simulink model "MDCC_DeadComp"  (R2023a)
settings: Solver=FixedStepDiscrete  StartTime=0.0  StopTime=10.0  FixedStep=0.0001  RelTol=1e-3
model workspace (MATLAB code in the model file):
  | cmdLim = Simulink.Parameter;
  | cmdLim.Value = 15;
  | cmdLim.Description = 'Limit for controlling the maximum surface command angle.';
  | cmdLim.Min = 0;
  | cmdLim.Max = 90;
  | cmdLim.DocUnits = 'deg';
  | 
  | dispGain = Simulink.Parameter;
  | dispGain.Value = 0.75;
  | dispGain.Description = 'Gain applied to the displacement error.';
  | dispGain.Min = 0;
  | dispGain.Max = [];
  | dispGain.DocUnits = 'deg/sec/deg';
  | 
  | dispLim = Simulink.Parameter;
  | dispLim.Value = 30;
  | dispLim.Description = 'Limit for controlling the maximum commanded angle.';
  | dispLim.Min = 0;
  | dispLim.Max = 180;
  | dispLim.DocUnits = 'deg';
  | 
  | intGain = Simulink.Parameter;
  | intGain.Value = 0.5;
  | intGain.Description = 'Gain applied to the integral error.';
  | intGain.Min = 0;
  | intGain.Max = [];
  | intGain.DocUnits = 'deg/sec/deg/sec';
  | 
  | intLim = Simulink.Parameter;
  | intLim.Value = 5;
  | intLim.Description = 'Limit for controlling the maximum commanded angle.';
  | intLim.Min = 0;
  | intLim.Max = 90;
  | intLim.DocUnits = 'deg';
  | 
  | rateGain = Simulink.Parameter;
  | rateGain.Value = 2;
  | rateGain.Description = 'Gain applied to the rate error.';
  | rateGain.Min = 0;
  | rateGain.Max = [];
  | rateGain.DocUnits = 'deg/deg/sec';
  | 
  | rateLim = Simulink.Parameter;
  | rateLim.Value = 6;
  | rateLim.Description = 'Limit for controlling the maximum commanded angle.';
  | rateLim.Min = 0;
  | rateLim.Max = 180;
  | rateLim.DocUnits = 'deg/sec';
  | 
  | hdgGain = Simulink.Parameter;
  | hdgGain.Value = 0.015;
values from neighbouring files (symbols this model uses):
  Ts = 5E-6    (= 5e-06)    [iPMSM_data.m]
undefined symbols (not defined in the file or in its folder): CosTable12bit_Y, GLBCal_GLBCal_Kf_DCLinkOverVolErrThd_V, GLBCal_GLBCal_Kf_DCLinkUnderVolErrThd_V, GLBCal_GLBCal_Kf_EquiLd_NULL, GLBCal_GLBCal_Kf_EquiLq_NULL, GLBCal_GLBCal_Kf_MotorRatedSpeed_rpm, GLBCal_GLBCal_Kf_MotorSpeedHysteresis_Coef, GLBCal_Ke_MotorPolePairsNum_NULL, IoHwAbOpArg_PwmDutyCyclePhU_NULL, IoHwAbOpArg_PwmDutyCyclePhV_NULL, IoHwAbOpArg_PwmDutyCyclePhW_NULL, IoHwAbOpArg_PwmOutputEn, KbMDCC_DeadTimeCompEn_flg, KbMDCC_MCF_flgHarmInject_flg, KbMDCC_SetEAngleEn_flg, KbMDCC_UdUqFwOmit_flg, KfMDCC_AbsIs_A, KfMDCC_ActiveDischargeIdCurVal_A, KfMDCC_ActiveDischargeIqCurVal_A, KfMDCC_DCLinkVolRate_coef, KfMDCC_DeadRate_NULL, KfMDCC_DebugEAngleInit_rad, KfMDCC_DebugUalphaVolCmd_V, KfMDCC_DebugUbetaVolCmd_V, KfMDCC_DebugUdCmd_V, KfMDCC_DebugUqCmd_V, KfMDCC_DebugUsCmd_V, KfMDCC_DebugUsRate_V, KfMDCC_Duty_Coef, KfMDCC_IMCResp_NULL, KfMDCC_IMCStab_NULL, KfMDCC_InvParkCpPeriodTimesT_NULL, KfMDCC_MCF_Harm1113FLParamSpeedThrd_rads, KfMDCC_MCF_Harm57FLParamSpeedThrd_rads, KfMDCC_MCF_HarmCpnAg_NULL, KfMDCC_MCF_HarmfLParaHigh_coef, KfMDCC_MCF_HarmfLParaLow_coef, KfMDCC_MCF_HarmInSpdLimt_rpm, KfMDCC_MCF_HarmInUAlphaMax_V, KfMDCC_MCF_HarmInUbetaMax_V, KfMDCC_MotorSpeedRadsDAQFactor_NULL, KfMDCC_ResScal_Coef, KfMDCC_SelfHeatingUdVal_V, KfMDCC_SelfHeatingUdValRate_V, KfMDCC_SpdIMCResp_rpm, KfMDCC_SpdIMCStab_rpm, KfMDCC_VfMDCC_DCLinkCurValFactor_NULL, KfMDCM_DCLinkCoef, KfMDCM_DCLinkRatedVoltage_V, KfMDCM_FluxWeakningVolFWOffset_V, KuMDCC_PositionResolution_NULL, KuMDCC_SetEAngle_Null, MDSM_MCUStatus, PiIoHwSetInvState_C_Sws_UVW_PwmEnOutput, PiIoHwSetInvState_C_SwsSet_DPO_UVW_Asc, PiIoHwSetInvState_C_SwsSet_DPO_UVW_FW, PiIoHwSetPwmDuty_C_SwsSet_DPO_UVW_Duty, SinTable12bit_Y, SVPWM, VfMDCC_DeadComSpeedHigh_Rpm ... (+5)
libraries: simulink x14, PMSM_Library x4
(part 5 of 6)

== system MDCC_DeadComp/DoCurCtr_sys/MDCC/UdUqCalc_Sys/MDCC_MCF_Sys1/Enabled Subsystem/Subsystem1/Park11/Subsystem1 ==
  dB_Harm : Inport
  MCF_dtPWM : Inport  Port=2
  In1 : Inport  Port=3
  Add : Sum
  Add1 : Sum  Inputs=-+
  Add2 : Sum
  Constant1 : Constant  OutDataTypeStr=single
  Constant2 : Constant  Value=2*pi  OutDataTypeStr=single
  Constant4 : Constant  OutDataTypeStr=single
  Divide{,1..3} (4 alike) : Product  Inputs=**
  Divide4 : Product  Inputs=*/
  Unit Delay : UnitDelay  SampleTime=-1  HasFrameUpgradeWarning=on
  Out1 : Outport
  wires:
  Unit Delay/1 -> Divide/1
  Divide1/1 -> Add/2
  In1/1 -> Divide1/2
  Divide4/1 -> Add1/1, Divide/2
  Add2/1 -> Divide4/2
  Constant4/1 -> Divide4/1, Add2/1
  Divide3/1 -> Add2/2
  Divide2/1 -> Divide3/2
  dB_Harm/1 -> Divide3/1
  MCF_dtPWM/1 -> Divide2/2
  Constant2/1 -> Divide2/1
  Add1/1 -> Divide1/1
  Constant1/1 -> Add1/2
  Divide/1 -> Add/1
  Add/1 -> Unit Delay/1, Out1/1

== system MDCC_DeadComp/DoCurCtr_sys/MDCC/UdUqCalc_Sys/MDCC_MCF_Sys1/Enabled Subsystem/Subsystem1/Park13/Subsystem ==
  In1 : Inport
  MCF_dtPWM : Inport  Port=2
  dB_Harm : Inport  Port=3
  Add : Sum
  Add1 : Sum  Inputs=-+
  Add2 : Sum
  Constant1 : Constant  OutDataTypeStr=single
  Constant2 : Constant  Value=2*pi  OutDataTypeStr=single
  Constant4 : Constant  OutDataTypeStr=single
  Divide{,1..3} (4 alike) : Product  Inputs=**
  Divide4 : Product  Inputs=*/
  Unit Delay : UnitDelay  SampleTime=-1  HasFrameUpgradeWarning=on
  Out1 : Outport
  wires:
  Add/1 -> Out1/1, Unit Delay/1
  Divide/1 -> Add/1
  Constant1/1 -> Add1/2
  Add1/1 -> Divide1/1
  Constant2/1 -> Divide2/1
  MCF_dtPWM/1 -> Divide2/2
  dB_Harm/1 -> Divide3/1
  Divide2/1 -> Divide3/2
  Divide3/1 -> Add2/2
  Constant4/1 -> Add2/1, Divide4/1
  Add2/1 -> Divide4/2
  Divide4/1 -> Divide/2, Add1/1
  In1/1 -> Divide1/2
  Divide1/1 -> Add/2
  Unit Delay/1 -> Divide/1

== system MDCC_DeadComp/DoCurCtr_sys/MDCC/UdUqCalc_Sys/MDCC_MCF_Sys1/Enabled Subsystem/Subsystem1/Park13/Subsystem1 ==
  dB_Harm : Inport
  MCF_dtPWM : Inport  Port=2
  In1 : Inport  Port=3
  Add : Sum
  Add1 : Sum  Inputs=-+
  Add2 : Sum
  Constant1 : Constant  OutDataTypeStr=single
  Constant2 : Constant  Value=2*pi  OutDataTypeStr=single
  Constant4 : Constant  OutDataTypeStr=single
  Divide{,1..3} (4 alike) : Product  Inputs=**
  Divide4 : Product  Inputs=*/
  Unit Delay : UnitDelay  SampleTime=-1  HasFrameUpgradeWarning=on
  Out1 : Outport
  wires:
  Unit Delay/1 -> Divide/1
  Divide1/1 -> Add/2
  In1/1 -> Divide1/2
  Divide4/1 -> Add1/1, Divide/2
  Add2/1 -> Divide4/2
  Constant4/1 -> Divide4/1, Add2/1
  Divide3/1 -> Add2/2
  Divide2/1 -> Divide3/2
  dB_Harm/1 -> Divide3/1
  MCF_dtPWM/1 -> Divide2/2
  Constant2/1 -> Divide2/1
  Add1/1 -> Divide1/1
  Constant1/1 -> Add1/2
  Divide/1 -> Add/1
  Add/1 -> Unit Delay/1, Out1/1

== system MDCC_DeadComp/DoCurCtr_sys/MDCC/UdUqCalc_Sys/MDCC_MCF_Sys1/Enabled Subsystem/Subsystem1/Park5/Subsystem ==
  In1 : Inport
  MCF_dtPWM : Inport  Port=2
  dB_Harm : Inport  Port=3
  Add : Sum
  Add1 : Sum  Inputs=-+
  Add2 : Sum
  Constant1 : Constant  OutDataTypeStr=single
  Constant2 : Constant  Value=2*pi  OutDataTypeStr=single
  Constant4 : Constant  OutDataTypeStr=single
  Divide{,1..3} (4 alike) : Product  Inputs=**
  Divide4 : Product  Inputs=*/
  Unit Delay : UnitDelay  SampleTime=-1  HasFrameUpgradeWarning=on
  Out1 : Outport
  wires:
  Add/1 -> Out1/1, Unit Delay/1
  Divide/1 -> Add/1
  Constant1/1 -> Add1/2
  Add1/1 -> Divide1/1
  Constant2/1 -> Divide2/1
  MCF_dtPWM/1 -> Divide2/2
  dB_Harm/1 -> Divide3/1
  Divide2/1 -> Divide3/2
  Divide3/1 -> Add2/2
  Constant4/1 -> Add2/1, Divide4/1
  Add2/1 -> Divide4/2
  Divide4/1 -> Divide/2, Add1/1
  In1/1 -> Divide1/2
  Divide1/1 -> Add/2
  Unit Delay/1 -> Divide/1

== system MDCC_DeadComp/DoCurCtr_sys/MDCC/UdUqCalc_Sys/MDCC_MCF_Sys1/Enabled Subsystem/Subsystem1/Park5/Subsystem1 ==
  dB_Harm : Inport
  MCF_dtPWM : Inport  Port=2
  In1 : Inport  Port=3
  Add : Sum
  Add1 : Sum  Inputs=-+
  Add2 : Sum
  Constant1 : Constant  OutDataTypeStr=single
  Constant2 : Constant  Value=2*pi  OutDataTypeStr=single
  Constant4 : Constant  OutDataTypeStr=single
  Divide{,1..3} (4 alike) : Product  Inputs=**
  Divide4 : Product  Inputs=*/
  Unit Delay : UnitDelay  SampleTime=-1  HasFrameUpgradeWarning=on
  Out1 : Outport
  wires:
  Unit Delay/1 -> Divide/1
  Divide1/1 -> Add/2
  In1/1 -> Divide1/2
  Divide4/1 -> Add1/1, Divide/2
  Add2/1 -> Divide4/2
  Constant4/1 -> Divide4/1, Add2/1
  Divide3/1 -> Add2/2
  Divide2/1 -> Divide3/2
  dB_Harm/1 -> Divide3/1
  MCF_dtPWM/1 -> Divide2/2
  Constant2/1 -> Divide2/1
  Add1/1 -> Divide1/1
  Constant1/1 -> Add1/2
  Divide/1 -> Add/1
  Add/1 -> Unit Delay/1, Out1/1

== system MDCC_DeadComp/DoCurCtr_sys/MDCC/UdUqCalc_Sys/MDCC_MCF_Sys1/Enabled Subsystem/Subsystem1/Park7/Subsystem ==
  In1 : Inport
  MCF_dtPWM : Inport  Port=2
  dB_Harm : Inport  Port=3
  Add : Sum
  Add1 : Sum  Inputs=-+
  Add2 : Sum
  Constant1 : Constant  OutDataTypeStr=single
  Constant2 : Constant  Value=2*pi  OutDataTypeStr=single
  Constant4 : Constant  OutDataTypeStr=single
  Divide{,1..3} (4 alike) : Product  Inputs=**
  Divide4 : Product  Inputs=*/
  Unit Delay : UnitDelay  SampleTime=-1  HasFrameUpgradeWarning=on
  Out1 : Outport
  wires:
  Add/1 -> Out1/1, Unit Delay/1
  Divide/1 -> Add/1
  Constant1/1 -> Add1/2
  Add1/1 -> Divide1/1
  Constant2/1 -> Divide2/1
  MCF_dtPWM/1 -> Divide2/2
  dB_Harm/1 -> Divide3/1
  Divide2/1 -> Divide3/2
  Divide3/1 -> Add2/2
  Constant4/1 -> Add2/1, Divide4/1
  Add2/1 -> Divide4/2
  Divide4/1 -> Divide/2, Add1/1
  In1/1 -> Divide1/2
  Divide1/1 -> Add/2
  Unit Delay/1 -> Divide/1

== system MDCC_DeadComp/DoCurCtr_sys/MDCC/UdUqCalc_Sys/MDCC_MCF_Sys1/Enabled Subsystem/Subsystem1/Park7/Subsystem1 ==
  dB_Harm : Inport
  MCF_dtPWM : Inport  Port=2
  In1 : Inport  Port=3
  Add : Sum
  Add1 : Sum  Inputs=-+
  Add2 : Sum
  Constant1 : Constant  OutDataTypeStr=single
  Constant2 : Constant  Value=2*pi  OutDataTypeStr=single
  Constant4 : Constant  OutDataTypeStr=single
  Divide{,1..3} (4 alike) : Product  Inputs=**
  Divide4 : Product  Inputs=*/
  Unit Delay : UnitDelay  SampleTime=-1  HasFrameUpgradeWarning=on
  Out1 : Outport
  wires:
  Unit Delay/1 -> Divide/1
  Divide1/1 -> Add/2
  In1/1 -> Divide1/2
  Divide4/1 -> Add1/1, Divide/2
  Add2/1 -> Divide4/2
  Constant4/1 -> Divide4/1, Add2/1
  Divide3/1 -> Add2/2
  Divide2/1 -> Divide3/2
  dB_Harm/1 -> Divide3/1
  MCF_dtPWM/1 -> Divide2/2
  Constant2/1 -> Divide2/1
  Add1/1 -> Divide1/1
  Constant1/1 -> Add1/2
  Divide/1 -> Add/1
  Add/1 -> Unit Delay/1, Out1/1

== system MDCC_DeadComp/DoCurCtr_sys/MDCC/UdUqCalc_Sys/MDCC_MCF_Sys1/Enabled Subsystem/Subsystem1/Subsystem/LookUpEAngleCosSin1 ==
  VuMDCC_MotorPositionCnt_NULL : Inport  OutMin=[0]  OutMax=[4095]
  Constant2 : Constant  Value=CosTable12bit_Y
  Constant3 : Constant  Value=SinTable12bit_Y
  Direct Lookup Table (n-D) : LookupNDDirect  NumberOfTableDimensions=1  TableIsInput=on  Table=[4 5 6]  TableMax=[4096]
  Direct Lookup Table (n-D)1 : LookupNDDirect  NumberOfTableDimensions=1  TableIsInput=on  Table=[4 5 6]  TableMax=[4096]
  VfMDCC_EAngleSin_NULL : Outport
  VfMDCC_EAngleCos_NULL : Outport  Port=2
  wires:
  VuMDCC_MotorPositionCnt_NULL/1 -> Direct Lookup Table (n-D)/1, Direct Lookup Table (n-D)1/1
  Direct Lookup Table (n-D)/1 -> VfMDCC_EAngleSin_NULL/1
  Direct Lookup Table (n-D)1/1 -> VfMDCC_EAngleCos_NULL/1
  Constant2/1 -> Direct Lookup Table (n-D)1/2
  Constant3/1 -> Direct Lookup Table (n-D)/2

== system MDCC_DeadComp/DoCurCtr_sys/MDCC/UdUqCalc_Sys/MDCC_MCF_Sys1/Enabled Subsystem/Subsystem1/Subsystem/LookUpEAngleCosSin2 ==
  VuMDCC_MotorPositionCnt_NULL : Inport  OutMin=[0]  OutMax=[4095]
  Constant2 : Constant  Value=CosTable12bit_Y
  Constant3 : Constant  Value=SinTable12bit_Y
  Direct Lookup Table (n-D) : LookupNDDirect  NumberOfTableDimensions=1  TableIsInput=on  Table=[4 5 6]  TableMax=[4096]
  Direct Lookup Table (n-D)1 : LookupNDDirect  NumberOfTableDimensions=1  TableIsInput=on  Table=[4 5 6]  TableMax=[4096]
  VfMDCC_EAngleSin_NULL : Outport
  VfMDCC_EAngleCos_NULL : Outport  Port=2
  wires:
  Constant3/1 -> Direct Lookup Table (n-D)/2
  Constant2/1 -> Direct Lookup Table (n-D)1/2
  Direct Lookup Table (n-D)1/1 -> VfMDCC_EAngleCos_NULL/1
  Direct Lookup Table (n-D)/1 -> VfMDCC_EAngleSin_NULL/1
  VuMDCC_MotorPositionCnt_NULL/1 -> Direct Lookup Table (n-D)1/1, Direct Lookup Table (n-D)/1

== system MDCC_DeadComp/DoCurCtr_sys/MDCC/UdUqCalc_Sys/MDCC_MCF_Sys1/Enabled Subsystem/Subsystem1/Subsystem/LookUpEAngleCosSin3 ==
  VuMDCC_MotorPositionCnt_NULL : Inport  OutMin=[0]  OutMax=[4095]
  Constant2 : Constant  Value=CosTable12bit_Y
  Constant3 : Constant  Value=SinTable12bit_Y
  Direct Lookup Table (n-D) : LookupNDDirect  NumberOfTableDimensions=1  TableIsInput=on  Table=[4 5 6]  TableMax=[4096]
  Direct Lookup Table (n-D)1 : LookupNDDirect  NumberOfTableDimensions=1  TableIsInput=on  Table=[4 5 6]  TableMax=[4096]
  VfMDCC_EAngleSin_NULL : Outport
  VfMDCC_EAngleCos_NULL : Outport  Port=2
  wires:
  VuMDCC_MotorPositionCnt_NULL/1 -> Direct Lookup Table (n-D)/1, Direct Lookup Table (n-D)1/1
  Direct Lookup Table (n-D)/1 -> VfMDCC_EAngleSin_NULL/1
  Direct Lookup Table (n-D)1/1 -> VfMDCC_EAngleCos_NULL/1
  Constant2/1 -> Direct Lookup Table (n-D)1/2
  Constant3/1 -> Direct Lookup Table (n-D)/2

== system MDCC_DeadComp/DoCurCtr_sys/MDCC/UdUqCalc_Sys/MDCC_MCF_Sys1/Enabled Subsystem/Subsystem1/Subsystem/LookUpEAngleCosSin4 ==
  VuMDCC_MotorPositionCnt_NULL : Inport  OutMin=[0]  OutMax=[4095]
  Constant2 : Constant  Value=CosTable12bit_Y
  Constant3 : Constant  Value=SinTable12bit_Y
  Direct Lookup Table (n-D) : LookupNDDirect  NumberOfTableDimensions=1  TableIsInput=on  Table=[4 5 6]  TableMax=[4096]
  Direct Lookup Table (n-D)1 : LookupNDDirect  NumberOfTableDimensions=1  TableIsInput=on  Table=[4 5 6]  TableMax=[4096]
  VfMDCC_EAngleSin_NULL : Outport
  VfMDCC_EAngleCos_NULL : Outport  Port=2
  wires:
  Constant3/1 -> Direct Lookup Table (n-D)/2
  Constant2/1 -> Direct Lookup Table (n-D)1/2
  Direct Lookup Table (n-D)1/1 -> VfMDCC_EAngleCos_NULL/1
  Direct Lookup Table (n-D)/1 -> VfMDCC_EAngleSin_NULL/1
  VuMDCC_MotorPositionCnt_NULL/1 -> Direct Lookup Table (n-D)1/1, Direct Lookup Table (n-D)/1

== system MDCC_DeadComp/DoCurCtr_sys/MDCC/UdUqCalc_Sys/MDCC_MCF_Sys1/Enabled Subsystem/Subsystem2/Mcf_AgTranCalc1/LookUpEAngleCosSin2 ==
  VuMDCC_MotorPositionCnt_NULL : Inport  OutMin=[0]  OutMax=[4095]
  Constant2 : Constant  Value=CosTable12bit_Y
  Constant3 : Constant  Value=SinTable12bit_Y
  Direct Lookup Table (n-D) : LookupNDDirect  NumberOfTableDimensions=1  TableIsInput=on  Table=[4 5 6]  TableMax=[4096]
  Direct Lookup Table (n-D)1 : LookupNDDirect  NumberOfTableDimensions=1  TableIsInput=on  Table=[4 5 6]  TableMax=[4096]
  VfMDCC_EAngleSin_NULL : Outport
  VfMDCC_EAngleCos_NULL : Outport  Port=2
  wires:
  Constant2/1 -> Direct Lookup Table (n-D)1/2
  Constant3/1 -> Direct Lookup Table (n-D)/2
  Direct Lookup Table (n-D)1/1 -> VfMDCC_EAngleCos_NULL/1
  Direct Lookup Table (n-D)/1 -> VfMDCC_EAngleSin_NULL/1
  VuMDCC_MotorPositionCnt_NULL/1 -> Direct Lookup Table (n-D)1/1, Direct Lookup Table (n-D)/1

== system MDCC_DeadComp/DoCurCtr_sys/MDCC/UdUqCalc_Sys/MDCC_MCF_Sys1/Enabled Subsystem/Subsystem2/Mcf_AgTranCalc2/LookUpEAngleCosSin2 ==
  VuMDCC_MotorPositionCnt_NULL : Inport  OutMin=[0]  OutMax=[4095]
  Constant2 : Constant  Value=CosTable12bit_Y
  Constant3 : Constant  Value=SinTable12bit_Y
  Direct Lookup Table (n-D) : LookupNDDirect  NumberOfTableDimensions=1  TableIsInput=on  Table=[4 5 6]  TableMax=[4096]
  Direct Lookup Table (n-D)1 : LookupNDDirect  NumberOfTableDimensions=1  TableIsInput=on  Table=[4 5 6]  TableMax=[4096]
  VfMDCC_EAngleSin_NULL : Outport
  VfMDCC_EAngleCos_NULL : Outport  Port=2
  wires:
  VuMDCC_MotorPositionCnt_NULL/1 -> Direct Lookup Table (n-D)/1, Direct Lookup Table (n-D)1/1
  Direct Lookup Table (n-D)/1 -> VfMDCC_EAngleSin_NULL/1
  Direct Lookup Table (n-D)1/1 -> VfMDCC_EAngleCos_NULL/1
  Constant3/1 -> Direct Lookup Table (n-D)/2
  Constant2/1 -> Direct Lookup Table (n-D)1/2

== system MDCC_DeadComp/DoCurCtr_sys/MDCC/UdUqCalc_Sys/MDCC_MCF_Sys1/Enabled Subsystem/Subsystem2/Mcf_AgTranCalc3/LookUpEAngleCosSin2 ==
  VuMDCC_MotorPositionCnt_NULL : Inport  OutMin=[0]  OutMax=[4095]
  Constant2 : Constant  Value=CosTable12bit_Y
  Constant3 : Constant  Value=SinTable12bit_Y
  Direct Lookup Table (n-D) : LookupNDDirect  NumberOfTableDimensions=1  TableIsInput=on  Table=[4 5 6]  TableMax=[4096]
  Direct Lookup Table (n-D)1 : LookupNDDirect  NumberOfTableDimensions=1  TableIsInput=on  Table=[4 5 6]  TableMax=[4096]
  VfMDCC_EAngleSin_NULL : Outport
  VfMDCC_EAngleCos_NULL : Outport  Port=2
  wires:
  Constant2/1 -> Direct Lookup Table (n-D)1/2
  Constant3/1 -> Direct Lookup Table (n-D)/2
  Direct Lookup Table (n-D)1/1 -> VfMDCC_EAngleCos_NULL/1
  Direct Lookup Table (n-D)/1 -> VfMDCC_EAngleSin_NULL/1
  VuMDCC_MotorPositionCnt_NULL/1 -> Direct Lookup Table (n-D)1/1, Direct Lookup Table (n-D)/1

== system MDCC_DeadComp/DoCurCtr_sys/MDCC/UdUqCalc_Sys/MDCC_MCF_Sys1/Enabled Subsystem/Subsystem2/Mcf_AgTranCalc5/LookUpEAngleCosSin2 ==
  VuMDCC_MotorPositionCnt_NULL : Inport  OutMin=[0]  OutMax=[4095]
  Constant2 : Constant  Value=CosTable12bit_Y
  Constant3 : Constant  Value=SinTable12bit_Y
  Direct Lookup Table (n-D) : LookupNDDirect  NumberOfTableDimensions=1  TableIsInput=on  Table=[4 5 6]  TableMax=[4096]
  Direct Lookup Table (n-D)1 : LookupNDDirect  NumberOfTableDimensions=1  TableIsInput=on  Table=[4 5 6]  TableMax=[4096]
  VfMDCC_EAngleSin_NULL : Outport
  VfMDCC_EAngleCos_NULL : Outport  Port=2
  wires:
  VuMDCC_MotorPositionCnt_NULL/1 -> Direct Lookup Table (n-D)/1, Direct Lookup Table (n-D)1/1
  Direct Lookup Table (n-D)/1 -> VfMDCC_EAngleSin_NULL/1
  Direct Lookup Table (n-D)1/1 -> VfMDCC_EAngleCos_NULL/1
  Constant3/1 -> Direct Lookup Table (n-D)/2
  Constant2/1 -> Direct Lookup Table (n-D)1/2

== system MDCC_DeadComp/DoCurCtr_sys/MDCC/SVM_Calc/MDSA/SVPWM1/vIntp_PWMFOC_CalTriCompValue/CalTabc/Cal_T1T2/Sec1 ==
  Bus_XYZ_IN : Inport
  Action Port : ActionPort
  Bus Creator1 : BusCreator  Inputs=2
  Bus Selector : BusSelector  OutputSignals=Z,Y
  Signal Conversion : SignalConversion  OverrideOpt=off
  Signal Conversion1 : SignalConversion  OverrideOpt=off
  Bus_T1T2 : Outport
  wires:
  Bus Creator1/1 -> Bus_T1T2/1
  Bus_XYZ_IN/1 -> Bus Selector/1
  Bus Selector/1 -> Signal Conversion/1  "<Z>"
  Bus Selector/2 -> Signal Conversion1/1  "<Y>"
  Signal Conversion/1 -> Bus Creator1/1
  Signal Conversion1/1 -> Bus Creator1/2

== system MDCC_DeadComp/DoCurCtr_sys/MDCC/SVM_Calc/MDSA/SVPWM1/vIntp_PWMFOC_CalTriCompValue/CalTabc/Cal_T1T2/Sec2 ==
  Bus_XYZ_IN : Inport
  Action Port : ActionPort
  -1 : Constant  Value=-1
  Bus Creator1 : BusCreator  Inputs=2
  Bus Selector : BusSelector  OutputSignals=Y,X
  Data Type Conversion1 : DataTypeConversion  SaturateOnIntegerOverflow=off  RndMeth=Floor
  Product1 : Product
  Signal Conversion1 : SignalConversion  OverrideOpt=off
  Bus_T1T2 : Outport
  wires:
  -1/1 -> Data Type Conversion1/1
  Data Type Conversion1/1 -> Product1/2
  Product1/1 -> Bus Creator1/2
  Bus Creator1/1 -> Bus_T1T2/1
  Bus Selector/2 -> Product1/1  "<X>"
  Bus Selector/1 -> Signal Conversion1/1  "<Y>"
  Bus_XYZ_IN/1 -> Bus Selector/1
  Signal Conversion1/1 -> Bus Creator1/1

== system MDCC_DeadComp/DoCurCtr_sys/MDCC/SVM_Calc/MDSA/SVPWM1/vIntp_PWMFOC_CalTriCompValue/CalTabc/Cal_T1T2/Sec3 ==
  Bus_XYZ_IN : Inport
  Action Port : ActionPort
  -1 : Constant  Value=-1
  Bus Creator1 : BusCreator  Inputs=2
  Bus Selector : BusSelector  OutputSignals=Z,X
  Data Type Conversion1 : DataTypeConversion  SaturateOnIntegerOverflow=off  RndMeth=Floor
  Product1 : Product
  Signal Conversion1 : SignalConversion  OverrideOpt=off
  Bus_T1T2 : Outport
  wires:
  Bus Selector/2 -> Signal Conversion1/1  "<X>"
  -1/1 -> Data Type Conversion1/1
  Bus Selector/1 -> Product1/2  "<Z>"
  Product1/1 -> Bus Creator1/1
  Bus Creator1/1 -> Bus_T1T2/1
  Bus_XYZ_IN/1 -> Bus Selector/1
  Data Type Conversion1/1 -> Product1/1
  Signal Conversion1/1 -> Bus Creator1/2

== system MDCC_DeadComp/DoCurCtr_sys/MDCC/SVM_Calc/MDSA/SVPWM1/vIntp_PWMFOC_CalTriCompValue/CalTabc/Cal_T1T2/Sec4 ==
  Bus_XYZ_IN : Inport
  Action Port : ActionPort
  -1 : Constant  Value=-1
  Bus Creator1 : BusCreator  Inputs=2
  Bus Selector : BusSelector  OutputSignals=X,Z
  Data Type Conversion2 : DataTypeConversion  SaturateOnIntegerOverflow=off  RndMeth=Floor
  Product1 : Product
  Signal Conversion1 : SignalConversion  OverrideOpt=off
  Bus_T1T2 : Outport
  wires:
  -1/1 -> Data Type Conversion2/1
  Bus Selector/1 -> Product1/2  "<X>"
  Product1/1 -> Bus Creator1/1
  Bus Creator1/1 -> Bus_T1T2/1
  Bus Selector/2 -> Signal Conversion1/1  "<Z>"
  Bus_XYZ_IN/1 -> Bus Selector/1
  Data Type Conversion2/1 -> Product1/1
  Signal Conversion1/1 -> Bus Creator1/2

== system MDCC_DeadComp/DoCurCtr_sys/MDCC/SVM_Calc/MDSA/SVPWM1/vIntp_PWMFOC_CalTriCompValue/CalTabc/Cal_T1T2/Sec5 ==
  Bus_XYZ_IN : Inport
  Action Port : ActionPort
  -1 : Constant  Value=-1
  Bus Creator1 : BusCreator  Inputs=2
  Bus Selector : BusSelector  OutputSignals=X,Y
  Data Type Conversion1 : DataTypeConversion  SaturateOnIntegerOverflow=off  RndMeth=Floor
  Product1 : Product
  Signal Conversion1 : SignalConversion  OverrideOpt=off
  Bus_T1T2 : Outport
  wires:
  Bus Selector/1 -> Signal Conversion1/1  "<X>"
  Bus Selector/2 -> Product1/1  "<Y>"
  -1/1 -> Data Type Conversion1/1
  Data Type Conversion1/1 -> Product1/2
  Product1/1 -> Bus Creator1/2
  Bus Creator1/1 -> Bus_T1T2/1
  Bus_XYZ_IN/1 -> Bus Selector/1
  Signal Conversion1/1 -> Bus Creator1/1

== system MDCC_DeadComp/DoCurCtr_sys/MDCC/SVM_Calc/MDSA/SVPWM1/vIntp_PWMFOC_CalTriCompValue/CalTabc/Cal_T1T2/Sec6 ==
  Bus_XYZ_IN : Inport
  Action Port : ActionPort
  -1 : Constant  Value=-1
  -1_1 : Constant  Value=-1
  Bus Creator1 : BusCreator  Inputs=2
  Bus Selector : BusSelector  OutputSignals=Y,Z
  Data Type Conversion2 : DataTypeConversion  SaturateOnIntegerOverflow=off  RndMeth=Floor
  Data Type Conversion3 : DataTypeConversion  SaturateOnIntegerOverflow=off  RndMeth=Floor
  Product2 : Product
  Product3 : Product
  Bus_T1T2 : Outport
  wires:
  Bus Selector/2 -> Product2/1  "<Z>"
  Bus Selector/1 -> Product3/2  "<Y>"
  -1/1 -> Data Type Conversion3/1
  -1_1/1 -> Data Type Conversion2/1
  Data Type Conversion2/1 -> Product2/2
  Product2/1 -> Bus Creator1/2
  Product3/1 -> Bus Creator1/1
  Bus Creator1/1 -> Bus_T1T2/1
  Bus_XYZ_IN/1 -> Bus Selector/1
  Data Type Conversion3/1 -> Product3/1

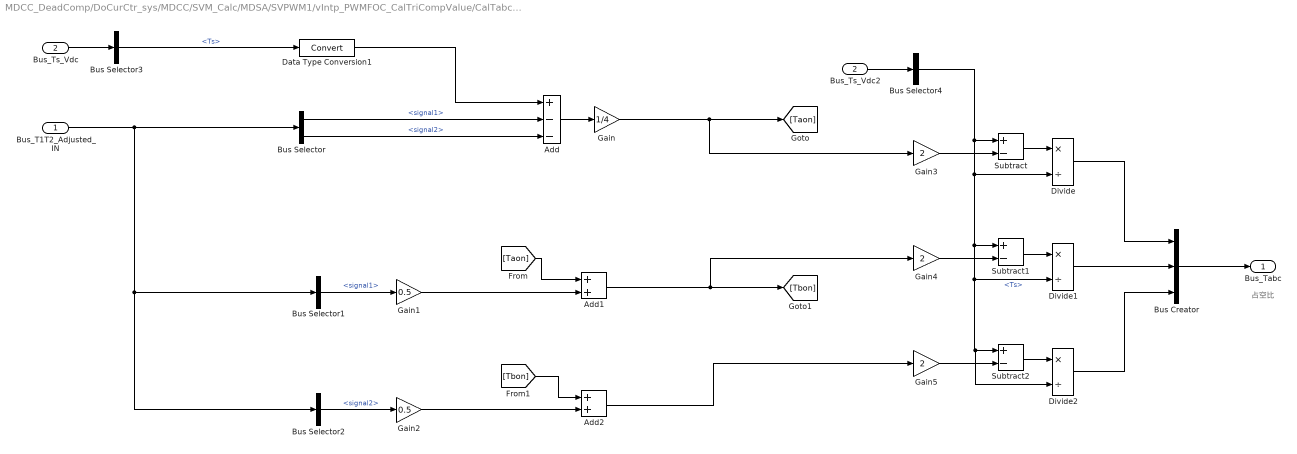
== system MDCC_DeadComp/DoCurCtr_sys/MDCC/SVM_Calc/MDSA/SVPWM1/vIntp_PWMFOC_CalTriCompValue/CalTabc/Cal_TabcValue/CalTabcValue ==
  note: 占空比
  Bus_T1T2_Adjusted_IN : Inport
  Bus_Ts_Vdc : Inport  Port=2
  Add : Sum  Inputs=+--
  Add1 : Sum
  Add2 : Sum
  Bus Creator : BusCreator  Inputs=3
  Bus Selector : BusSelector  OutputSignals=signal1,signal2
  Bus Selector1 : BusSelector  OutputSignals=signal1
  Bus Selector2 : BusSelector  OutputSignals=signal2
  Bus Selector3 : BusSelector  OutputSignals=Ts
  Bus Selector4 : BusSelector  OutputSignals=Ts
  Bus_Ts_Vdc2 : InportShadow  Port=2
  Data Type Conversion1 : DataTypeConversion  SaturateOnIntegerOverflow=off  RndMeth=Floor
  Divide : Product  Inputs=*/
  Divide1 : Product  Inputs=*/
  Divide2 : Product  Inputs=*/
  Gain : Gain  Gain=1/4
  Gain1 : Gain  Gain=0.5
  Gain2 : Gain  Gain=0.5
  Gain3 : Gain  Gain=2
  Gain4 : Gain  Gain=2
  Gain5 : Gain  Gain=2
  Subtract : Sum  Inputs=+-
  Subtract1 : Sum  Inputs=+-
  Subtract2 : Sum  Inputs=+-
  Bus_Tabc : Outport  Description=高电平计数值
  wires:
  Bus_Ts_Vdc2/1 -> Bus Selector4/1
  Bus_Ts_Vdc/1 -> Bus Selector3/1
  Divide2/1 -> Bus Creator/3
  Divide/1 -> Bus Creator/1
  Divide1/1 -> Bus Creator/2
  Subtract2/1 -> Divide2/1
  Subtract/1 -> Divide/1
  Subtract1/1 -> Divide1/1
  Bus Selector4/1 -> Subtract/1, Divide/2, Divide1/2, Subtract2/1, Divide2/2, Subtract1/1  "<Ts>"
  Gain5/1 -> Subtract2/2
  Gain4/1 -> Subtract1/2
  Gain3/1 -> Subtract/2
  Add2/1 -> Gain5/1
  Add1/1 -> [Tbon], Gain4/1
  Gain2/1 -> Add2/2
  Gain1/1 -> Add1/2
  Gain/1 -> [Taon], Gain3/1
  Data Type Conversion1/1 -> Add/1
  Bus_T1T2_Adjusted_IN/1 -> Bus Selector2/1, Bus Selector1/1, Bus Selector/1
  Bus Selector3/1 -> Data Type Conversion1/1  "<Ts>"
  Bus Selector/1 -> Add/2  "<signal1>"
  Bus Selector/2 -> Add/3  "<signal2>"
  Add/1 -> Gain/1
  Bus Selector1/1 -> Gain1/1  "<signal1>"
  [Taon] -> Add1/1
  Bus Selector2/1 -> Gain2/1  "<signal2>"
  [Tbon] -> Add2/1
  Bus Creator/1 -> Bus_Tabc/1

== system MDCC_DeadComp/DoCurCtr_sys/MDCC/SVM_Calc/MDSA/SVPWM1/vIntp_PWMFOC_CalTriCompValue/CalTabc/Cal_TabcValue/ManageT1T2 ==
  Bus_T1T2_IN : Inport
  Bus_Ts_Vdc : Inport  Port=2
  Add : Sum
  Bus Creator : BusCreator  Inputs=2
  Bus Selector : BusSelector  OutputSignals=signal1,signal2
  Bus Selector1 : BusSelector  OutputSignals=signal1,signal2
  Bus Selector2 : BusSelector  OutputSignals=signal1,signal2
  Bus Selector3 : BusSelector  OutputSignals=Ts
  Constant1 : Constant
  Data Type Conversion : DataTypeConversion  SaturateOnIntegerOverflow=off  RndMeth=Floor
  Data Type Conversion1 : DataTypeConversion  SaturateOnIntegerOverflow=off  RndMeth=Floor
  Divide : Product  Inputs=*/
  Relational Operator : RelationalOperator  Operator=>  OutDataTypeStr=boolean  InputSameDT=off
  Signal Conversion : SignalConversion  OverrideOpt=off
  Signal Conversion1 : SignalConversion  OverrideOpt=off
  Subsystem : Subsystem
  Switch : Switch  Criteria=u2 ~= 0  OutDataTypeStr=single  ZeroCross=off  SaturateOnIntegerOverflow=off  InputSameDT=off
  Switch1 : Switch  Criteria=u2 ~= 0  OutDataTypeStr=single  ZeroCross=off  SaturateOnIntegerOverflow=off  InputSameDT=off
  Bus_T1T2_Adjusted : Outport
  wires:
  [Bus_Ts_Vdc_ManageT1T2] -> Subsystem/2(Bus_Ts_Vdc)
  Bus Selector3/1 -> Data Type Conversion1/1  "<Ts>"
  [Bus_Ts_Vdc_ManageT1T2] -> Bus Selector3/1
  Bus_Ts_Vdc/1 -> [Bus_Ts_Vdc_ManageT1T2]
  Bus Creator/1 -> Bus_T1T2_Adjusted/1
  Switch1/1 -> Bus Creator/2
  Bus Selector1/2 -> Switch1/3  "<signal2>"
  Bus Selector2/2 -> Switch1/1  "<signal2>"
  Switch/1 -> Bus Creator/1
  Bus Selector2/1 -> Switch/1  "<signal1>"
  Bus Selector1/1 -> Switch/3  "<signal1>"
  Subsystem/1(Out1) -> Bus Selector2/1
  Signal Conversion/1 -> Bus Selector1/1
  Signal Conversion1/1 -> Subsystem/1(Bus_T1T2_IN)
  Bus_T1T2_IN/1 -> Signal Conversion1/1, Bus Selector/1, Signal Conversion/1
  Bus Selector/1 -> Add/1  "<signal1>"
  Bus Selector/2 -> Add/2  "<signal2>"
  Constant1/1 -> Data Type Conversion/1
  Data Type Conversion/1 -> Divide/2
  Data Type Conversion1/1 -> Divide/1
  Add/1 -> Relational Operator/1
  Divide/1 -> Relational Operator/2
  Relational Operator/1 -> Switch/2, Switch1/2

== system MDCC_DeadComp/DoCurCtr_sys/MDCC/UdUqCalc_Sys/MDCC_MCF_Sys1/Enabled Subsystem/Harmonic_Injection_11/Subsystem/Harm_11Step_KpKi/Harm_11Step_daxis_PI ==
  MCF_Harm_isdDes11 : Inport
  MCF_Harm_isdAct11 : Inport  Port=2
  MCF_Harm_Kp : Inport  Port=3
  MCF_Harm_Ki : Inport  Port=4
  MCF_flgHarm11PIRest : Inport  Port=5
  Add : Sum  Inputs=+-
  Add1 : Sum  Inputs=+-
  Add2 : Sum  Inputs=+++
  Constant : Constant  Value=0  OutDataTypeStr=single
  Constant1 : Constant  Value=KfMDCM_DCLinkRatedVoltage_V*KfMDCM_DCLinkCoef*-1
  Constant3 : Constant  Value=KfMDCM_DCLinkRatedVoltage_V*KfMDCM_DCLinkCoef
  Product : Product
  Product1 : Product
  Saturation : simulink/Discontinuities/Saturation Dynamic  OutMin=[]  OutMax=[]  OutDataTypeStr=Inherit: Same as second input  OutDataType=fixdt(1, 16)  OutScaling=2^-10  DoSatur=off
      link override Data Type Propagation: ValuesUsedBestPrec=[11 -11]
  Switch : Switch  Criteria=u2 ~= 0  SaturateOnIntegerOverflow=off  InputSameDT=off
  Unit Delay : UnitDelay  SampleTime=-1  HasFrameUpgradeWarning=on
  Unit Delay1 : UnitDelay  SampleTime=-1  HasFrameUpgradeWarning=on
  MCF_Harm_ud11PI : Outport  VectorParamsAs1DForOutWhenUnconnected=off
  wires:
  MCF_Harm_isdAct11/1 -> Add/2
  MCF_Harm_isdDes11/1 -> Add/1
  MCF_Harm_Ki/1 -> Product1/2
  Switch/1 -> Add2/3
  Product/1 -> Add2/1
  Product1/1 -> Add2/2
  MCF_Harm_Kp/1 -> Product/2
  Add1/1 -> Product/1
  Unit Delay/1 -> Add1/2
  Add/1 -> Add1/1, Unit Delay/1, Product1/1
  Add2/1 -> Saturation/2
  Saturation/1 -> Unit Delay1/1, MCF_Harm_ud11PI/1
  Constant3/1 -> Saturation/1
  Constant1/1 -> Saturation/3
  MCF_flgHarm11PIRest/1 -> Switch/2
  Constant/1 -> Switch/3
  Unit Delay1/1 -> Switch/1

== system MDCC_DeadComp/DoCurCtr_sys/MDCC/UdUqCalc_Sys/MDCC_MCF_Sys1/Enabled Subsystem/Harmonic_Injection_11/Subsystem/Harm_11Step_KpKi/Harm_11Step_qaxis_PI ==
  MCF_Harm_isqDes11 : Inport
  MCF_Harm_isqAct11 : Inport  Port=2
  MCF_Harm_Kp : Inport  Port=3
  MCF_Harm_Ki : Inport  Port=4
  MCF_flgHarm11PIRest : Inport  Port=5
  Add : Sum  Inputs=+-
  Add1 : Sum  Inputs=+-
  Add2 : Sum  Inputs=+++
  Constant : Constant  Value=0  OutDataTypeStr=single
  Constant1 : Constant  Value=KfMDCM_DCLinkRatedVoltage_V*KfMDCM_DCLinkCoef*-1
  Constant3 : Constant  Value=KfMDCM_DCLinkRatedVoltage_V*KfMDCM_DCLinkCoef
  Product : Product
  Product1 : Product
  Saturation : simulink/Discontinuities/Saturation Dynamic  OutMin=[]  OutMax=[]  OutDataTypeStr=Inherit: Same as second input  OutDataType=fixdt(1, 16)  OutScaling=2^-10  DoSatur=off
      link override Data Type Propagation: ValuesUsedBestPrec=[11 -11]
  Switch : Switch  Criteria=u2 ~= 0  SaturateOnIntegerOverflow=off  InputSameDT=off
  Unit Delay : UnitDelay  SampleTime=-1  HasFrameUpgradeWarning=on
  Unit Delay2 : UnitDelay  SampleTime=-1  HasFrameUpgradeWarning=on
  MCF_Harm_uq11PI : Outport  VectorParamsAs1DForOutWhenUnconnected=off
  wires:
  Add/1 -> Product1/1, Unit Delay/1, Add1/1
  Unit Delay/1 -> Add1/2
  Add1/1 -> Product/1
  MCF_Harm_Kp/1 -> Product/2
  Product1/1 -> Add2/2
  Product/1 -> Add2/1
  MCF_Harm_Ki/1 -> Product1/2
  MCF_Harm_isqDes11/1 -> Add/1
  MCF_Harm_isqAct11/1 -> Add/2
  Constant1/1 -> Saturation/3
  Add2/1 -> Saturation/2
  Constant3/1 -> Saturation/1
  MCF_flgHarm11PIRest/1 -> Switch/2
  Saturation/1 -> Unit Delay2/1, MCF_Harm_uq11PI/1
  Switch/1 -> Add2/3
  Constant/1 -> Switch/3
  Unit Delay2/1 -> Switch/1

== system MDCC_DeadComp/DoCurCtr_sys/MDCC/UdUqCalc_Sys/MDCC_MCF_Sys1/Enabled Subsystem/Harmonic_Injection_13/Subsystem/Harm_13Step_KpKi/Harm_13Step_daxis_PI ==
  MCF_Harm_isdDes13 : Inport
  MCF_Harm_isdAct13 : Inport  Port=2
  MCF_Harm_Kp : Inport  Port=3
  MCF_Harm_Ki : Inport  Port=4
  MCF_flgHarm13PIRest : Inport  Port=5
  Add : Sum  Inputs=+-
  Add1 : Sum  Inputs=+-
  Add2 : Sum  Inputs=+++
  Constant : Constant  Value=0  OutDataTypeStr=single
  Constant1 : Constant  Value=KfMDCM_DCLinkRatedVoltage_V*KfMDCM_DCLinkCoef*-1
  Constant3 : Constant  Value=KfMDCM_DCLinkRatedVoltage_V*KfMDCM_DCLinkCoef
  Product : Product
  Product1 : Product
  Saturation : simulink/Discontinuities/Saturation Dynamic  OutMin=[]  OutMax=[]  OutDataTypeStr=Inherit: Same as second input  OutDataType=fixdt(1, 16)  OutScaling=2^-10  DoSatur=off
      link override Data Type Propagation: ValuesUsedBestPrec=[13 -13]
  Switch : Switch  Criteria=u2 ~= 0  SaturateOnIntegerOverflow=off  InputSameDT=off
  Unit Delay : UnitDelay  SampleTime=-1  HasFrameUpgradeWarning=on
  Unit Delay1 : UnitDelay  SampleTime=-1  HasFrameUpgradeWarning=on
  MCF_Harm_ud13PI : Outport  VectorParamsAs1DForOutWhenUnconnected=off
  wires:
  MCF_Harm_isdAct13/1 -> Add/2
  MCF_Harm_isdDes13/1 -> Add/1
  MCF_Harm_Ki/1 -> Product1/2
  Switch/1 -> Add2/3
  Product/1 -> Add2/1
  Product1/1 -> Add2/2
  MCF_Harm_Kp/1 -> Product/2
  Add1/1 -> Product/1
  Unit Delay/1 -> Add1/2
  Add/1 -> Add1/1, Unit Delay/1, Product1/1
  Add2/1 -> Saturation/2
  Saturation/1 -> Unit Delay1/1, MCF_Harm_ud13PI/1
  Constant3/1 -> Saturation/1
  Constant1/1 -> Saturation/3
  MCF_flgHarm13PIRest/1 -> Switch/2
  Constant/1 -> Switch/3
  Unit Delay1/1 -> Switch/1

== system MDCC_DeadComp/DoCurCtr_sys/MDCC/UdUqCalc_Sys/MDCC_MCF_Sys1/Enabled Subsystem/Harmonic_Injection_13/Subsystem/Harm_13Step_KpKi/Harm_13Step_qaxis_PI ==
  MCF_Harm_isqDes13 : Inport
  MCF_Harm_isqAct13 : Inport  Port=2
  MCF_Harm_Kp : Inport  Port=3
  MCF_Harm_Ki : Inport  Port=4
  MCF_flgHarm13PIRest : Inport  Port=5
  Add : Sum  Inputs=+-
  Add1 : Sum  Inputs=+-
  Add2 : Sum  Inputs=+++
  Constant : Constant  Value=0  OutDataTypeStr=single
  Constant1 : Constant  Value=KfMDCM_DCLinkRatedVoltage_V*KfMDCM_DCLinkCoef*-1
  Constant3 : Constant  Value=KfMDCM_DCLinkRatedVoltage_V*KfMDCM_DCLinkCoef
  Product : Product
  Product1 : Product
  Saturation : simulink/Discontinuities/Saturation Dynamic  OutMin=[]  OutMax=[]  OutDataTypeStr=Inherit: Same as second input  OutDataType=fixdt(1, 16)  OutScaling=2^-10  DoSatur=off
      link override Data Type Propagation: ValuesUsedBestPrec=[13 -13]
  Switch : Switch  Criteria=u2 ~= 0  SaturateOnIntegerOverflow=off  InputSameDT=off
  Unit Delay : UnitDelay  SampleTime=-1  HasFrameUpgradeWarning=on
  Unit Delay2 : UnitDelay  SampleTime=-1  HasFrameUpgradeWarning=on
  MCF_Harm_uq13PI : Outport  VectorParamsAs1DForOutWhenUnconnected=off
  wires:
  Add/1 -> Product1/1, Unit Delay/1, Add1/1
  Unit Delay/1 -> Add1/2
  Add1/1 -> Product/1
  MCF_Harm_Kp/1 -> Product/2
  Product1/1 -> Add2/2
  Product/1 -> Add2/1
  MCF_Harm_Ki/1 -> Product1/2
  MCF_Harm_isqDes13/1 -> Add/1
  MCF_Harm_isqAct13/1 -> Add/2
  Constant1/1 -> Saturation/3
  Add2/1 -> Saturation/2
  Constant3/1 -> Saturation/1
  MCF_flgHarm13PIRest/1 -> Switch/2
  Saturation/1 -> Unit Delay2/1, MCF_Harm_uq13PI/1
  Switch/1 -> Add2/3
  Constant/1 -> Switch/3
  Unit Delay2/1 -> Switch/1

== system MDCC_DeadComp/DoCurCtr_sys/MDCC/UdUqCalc_Sys/MDCC_MCF_Sys1/Enabled Subsystem/Harmonic_Injection_5/Subsystem/Harm_5Step_KpKi/Harm_5Step_daxis_PI ==
  MCF_Harm_isdDes5 : Inport
  MCF_Harm_isdAct5 : Inport  Port=2
  MCF_Harm_Kp : Inport  Port=3
  MCF_Harm_Ki : Inport  Port=4
  MCF_flgHarm5PIRest : Inport  Port=5
  Add : Sum  Inputs=+-
  Add1 : Sum  Inputs=+-
  Add2 : Sum  Inputs=+++
  Constant : Constant  Value=0  OutDataTypeStr=single
  Constant1 : Constant  Value=-1*KfMDCM_DCLinkRatedVoltage_V*KfMDCM_DCLinkCoef
  Constant3 : Constant  Value=KfMDCM_DCLinkRatedVoltage_V*KfMDCM_DCLinkCoef
  Product : Product
  Product1 : Product
  Saturation : simulink/Discontinuities/Saturation Dynamic  OutMin=[]  OutMax=[]  OutDataTypeStr=Inherit: Same as second input  OutDataType=fixdt(1, 16)  OutScaling=2^-10  DoSatur=off
  Switch : Switch  Criteria=u2 ~= 0  SaturateOnIntegerOverflow=off  InputSameDT=off
  Unit Delay : UnitDelay  SampleTime=-1  HasFrameUpgradeWarning=on
  Unit Delay1 : UnitDelay  SampleTime=-1  HasFrameUpgradeWarning=on
  MCF_Harm_ud5PI : Outport  VectorParamsAs1DForOutWhenUnconnected=off
  wires:
  MCF_Harm_isdAct5/1 -> Add/2
  MCF_Harm_isdDes5/1 -> Add/1
  MCF_Harm_Ki/1 -> Product1/2
  Switch/1 -> Add2/3
  Product/1 -> Add2/1
  Product1/1 -> Add2/2
  MCF_Harm_Kp/1 -> Product/2
  Add1/1 -> Product/1
  Unit Delay/1 -> Add1/2
  Add/1 -> Add1/1, Unit Delay/1, Product1/1
  Add2/1 -> Saturation/2
  Saturation/1 -> Unit Delay1/1, MCF_Harm_ud5PI/1
  Constant3/1 -> Saturation/1
  Constant1/1 -> Saturation/3
  MCF_flgHarm5PIRest/1 -> Switch/2
  Constant/1 -> Switch/3
  Unit Delay1/1 -> Switch/1

== system MDCC_DeadComp/DoCurCtr_sys/MDCC/UdUqCalc_Sys/MDCC_MCF_Sys1/Enabled Subsystem/Harmonic_Injection_5/Subsystem/Harm_5Step_KpKi/Harm_5Step_qaxis_PI ==
  MCF_Harm_isqDes5 : Inport
  MCF_Harm_isqAct5 : Inport  Port=2
  MCF_Harm_Kp : Inport  Port=3
  MCF_Harm_Ki : Inport  Port=4
  MCF_flgHarm5PIRest : Inport  Port=5
  Add : Sum  Inputs=+-
  Add1 : Sum  Inputs=+-
  Add2 : Sum  Inputs=+++
  Constant : Constant  Value=0  OutDataTypeStr=single
  Constant1 : Constant  Value=-1*KfMDCM_DCLinkRatedVoltage_V*KfMDCM_DCLinkCoef
  Constant3 : Constant  Value=KfMDCM_DCLinkRatedVoltage_V*KfMDCM_DCLinkCoef
  Product : Product
  Product1 : Product
  Saturation : simulink/Discontinuities/Saturation Dynamic  OutMin=[]  OutMax=[]  OutDataTypeStr=Inherit: Same as second input  OutDataType=fixdt(1, 16)  OutScaling=2^-10  DoSatur=off
  Switch : Switch  Criteria=u2 ~= 0  SaturateOnIntegerOverflow=off  InputSameDT=off
  Unit Delay : UnitDelay  SampleTime=-1  HasFrameUpgradeWarning=on
  Unit Delay2 : UnitDelay  SampleTime=-1  HasFrameUpgradeWarning=on
  MCF_Harm_uq5PI : Outport  VectorParamsAs1DForOutWhenUnconnected=off
  wires:
  Add/1 -> Product1/1, Unit Delay/1, Add1/1
  Unit Delay/1 -> Add1/2
  Add1/1 -> Product/1
  MCF_Harm_Kp/1 -> Product/2
  Product1/1 -> Add2/2
  Product/1 -> Add2/1
  MCF_Harm_Ki/1 -> Product1/2
  MCF_Harm_isqDes5/1 -> Add/1
  MCF_Harm_isqAct5/1 -> Add/2
  Constant1/1 -> Saturation/3
  Add2/1 -> Saturation/2
  Constant3/1 -> Saturation/1
  MCF_flgHarm5PIRest/1 -> Switch/2
  Saturation/1 -> Unit Delay2/1, MCF_Harm_uq5PI/1
  Switch/1 -> Add2/3
  Constant/1 -> Switch/3
  Unit Delay2/1 -> Switch/1

== system MDCC_DeadComp/DoCurCtr_sys/MDCC/UdUqCalc_Sys/MDCC_MCF_Sys1/Enabled Subsystem/Harmonic_Injection_7/Subsystem/Harm_7Step_KpKi/Harm_7Step_daxis_PI ==
  MCF_Harm_isdDes7 : Inport
  MCF_Harm_isdAct7 : Inport  Port=2
  MCF_Harm_Kp : Inport  Port=3
  MCF_Harm_Ki : Inport  Port=4
  MCF_flgHarm7PIRest : Inport  Port=5
  Add : Sum  Inputs=+-
  Add1 : Sum  Inputs=+-
  Add2 : Sum  Inputs=+++
  Constant : Constant  Value=0  OutDataTypeStr=single
  Constant1 : Constant  Value=-1*KfMDCM_DCLinkRatedVoltage_V*KfMDCM_DCLinkCoef
  Constant3 : Constant  Value=KfMDCM_DCLinkRatedVoltage_V*KfMDCM_DCLinkCoef
  Product : Product
  Product1 : Product
  Saturation : simulink/Discontinuities/Saturation Dynamic  OutMin=[]  OutMax=[]  OutDataTypeStr=Inherit: Same as second input  OutDataType=fixdt(1, 16)  OutScaling=2^-10  DoSatur=off
      link override Data Type Propagation: ValuesUsedBestPrec=[7 -7]
  Switch : Switch  Criteria=u2 ~= 0  SaturateOnIntegerOverflow=off  InputSameDT=off
  Unit Delay : UnitDelay  SampleTime=-1  HasFrameUpgradeWarning=on
  Unit Delay1 : UnitDelay  SampleTime=-1  HasFrameUpgradeWarning=on
  MCF_Harm_ud7PI : Outport  VectorParamsAs1DForOutWhenUnconnected=off
  wires:
  MCF_Harm_isdAct7/1 -> Add/2
  MCF_Harm_isdDes7/1 -> Add/1
  MCF_Harm_Ki/1 -> Product1/2
  Switch/1 -> Add2/3
  Product/1 -> Add2/1
  Product1/1 -> Add2/2
  MCF_Harm_Kp/1 -> Product/2
  Add1/1 -> Product/1
  Unit Delay/1 -> Add1/2
  Add/1 -> Add1/1, Unit Delay/1, Product1/1
  Add2/1 -> Saturation/2
  Saturation/1 -> Unit Delay1/1, MCF_Harm_ud7PI/1
  Constant3/1 -> Saturation/1
  Constant1/1 -> Saturation/3
  MCF_flgHarm7PIRest/1 -> Switch/2
  Constant/1 -> Switch/3
  Unit Delay1/1 -> Switch/1

== system MDCC_DeadComp/DoCurCtr_sys/MDCC/UdUqCalc_Sys/MDCC_MCF_Sys1/Enabled Subsystem/Harmonic_Injection_7/Subsystem/Harm_7Step_KpKi/Harm_7Step_qaxis_PI ==
  MCF_Harm_isqDes7 : Inport
  MCF_Harm_isqAct7 : Inport  Port=2
  MCF_Harm_Kp : Inport  Port=3
  MCF_Harm_Ki : Inport  Port=4
  MCF_flgHarm7PIRest : Inport  Port=5
  Add : Sum  Inputs=+-
  Add1 : Sum  Inputs=+-
  Add2 : Sum  Inputs=+++
  Constant : Constant  Value=0  OutDataTypeStr=single
  Constant1 : Constant  Value=-1*KfMDCM_DCLinkRatedVoltage_V*KfMDCM_DCLinkCoef
  Constant3 : Constant  Value=KfMDCM_DCLinkRatedVoltage_V*KfMDCM_DCLinkCoef
  Product : Product
  Product1 : Product
  Saturation : simulink/Discontinuities/Saturation Dynamic  OutMin=[]  OutMax=[]  OutDataTypeStr=Inherit: Same as second input  OutDataType=fixdt(1, 16)  OutScaling=2^-10  DoSatur=off
      link override Data Type Propagation: ValuesUsedBestPrec=[7 -7]
  Switch : Switch  Criteria=u2 ~= 0  SaturateOnIntegerOverflow=off  InputSameDT=off
  Unit Delay : UnitDelay  SampleTime=-1  HasFrameUpgradeWarning=on
  Unit Delay2 : UnitDelay  SampleTime=-1  HasFrameUpgradeWarning=on
  MCF_Harm_uq7PI : Outport  VectorParamsAs1DForOutWhenUnconnected=off
  wires:
  Add/1 -> Product1/1, Unit Delay/1, Add1/1
  Unit Delay/1 -> Add1/2
  Add1/1 -> Product/1
  MCF_Harm_Kp/1 -> Product/2
  Product1/1 -> Add2/2
  Product/1 -> Add2/1
  MCF_Harm_Ki/1 -> Product1/2
  MCF_Harm_isqDes7/1 -> Add/1
  MCF_Harm_isqAct7/1 -> Add/2
  Constant1/1 -> Saturation/3
  Add2/1 -> Saturation/2
  Constant3/1 -> Saturation/1
  MCF_flgHarm7PIRest/1 -> Switch/2
  Saturation/1 -> Unit Delay2/1, MCF_Harm_uq7PI/1
  Switch/1 -> Add2/3
  Constant/1 -> Switch/3
  Unit Delay2/1 -> Switch/1

== system MDCC_DeadComp/DoCurCtr_sys/MDCC/SVM_Calc/MDSA/SVPWM1/vIntp_PWMFOC_CalTriCompValue/CalTabc/Cal_TabcValue/ManageT1T2/Subsystem ==
  Bus_T1T2_IN : Inport
  Bus_Ts_Vdc : Inport  Port=2
  Add : Sum
  Bus Creator : BusCreator  Inputs=2
  Bus Selector : BusSelector  OutputSignals=signal1,signal2
  Bus Selector1 : BusSelector  OutputSignals=Ts
  Divide : Product  Inputs=*/
  Divide1 : Product  Inputs=*/
  Gain : Gain  Commented=on  Gain=Ts
  Gain1 : Gain  Commented=on  Gain=Ts
  Product : Product
  Product1 : Product
  Out1 : Outport
  wires:
  Product1/1 -> Bus Creator/1
  Divide/1 -> Product1/1
  Product/1 -> Bus Creator/2
  Divide1/1 -> Product/1
  Bus Selector1/1 -> Product/2, Product1/2  "<Ts>"
  Bus_Ts_Vdc/1 -> Bus Selector1/1
  Bus_T1T2_IN/1 -> Bus Selector/1
  Bus Selector/1 -> Divide/1, Add/1  "<signal1>"
  Bus Selector/2 -> [Bus_T1T2_T2], Add/2  "<signal2>"
  Add/1 -> Divide/2, Divide1/2
  [Bus_T1T2_T2] -> Divide1/1
  Bus Creator/1 -> Out1/1

== matlab function MDCC_DeadComp/DoCurCtr_sys/MDCC/UdUqCalc_Sys/UdUqCalc/IsDQCtl_m ==
  data: Decoup_coef input; PIReset input; TQC_UsdPI output; TQC_IsdDes input; TQC_IsqDes input; ISM_Isd input; ISM_Isq input; TQC_omSttr input; TQC_dtIsctl_Cc input; TQC_kidq input; TQC_kpd input; TQC_UsqPI output; TQC_kpq input; TQC_Rv input; TQC_UsqFluxExc input; TQC_uDaMax_Cc input; TQC_uQaMax_Cc input; facIntglDa_Dbg output; facIntglQa_Dbg output; facIntglDaQa_Dbg output; uDaUnlim_Dbg output; uQaUnlim_Dbg output; iDaDes_Dbg output; iQaDes_Dbg output
function [TQC_UsdPI,TQC_UsqPI,facIntglDa_Dbg,facIntglQa_Dbg,facIntglDaQa_Dbg,uDaUnlim_Dbg,uQaUnlim_Dbg,iDaDes_Dbg,iQaDes_Dbg] =fcn(Decoup_coef,PIReset,TQC_IsdDes,TQC_IsqDes,ISM_Isd,ISM_Isq,TQC_omSttr,TQC_dtIsctl_Cc,TQC_kidq,TQC_kpd,TQC_kpq,TQC_Rv,TQC_UsqFluxExc,TQC_uDaMax_Cc,TQC_uQaMax_Cc)

    persistent iDaDes iQaDes
    persistent iDaErrTust iQaErrTust
    persistent omSttr agDelta
    persistent facIntglDaQa facIntglDa facIntglQa
    persistent ydAdd yqAdd ydInt yqInt yPd yPq yRvd yRvq ydPFF yqPFF
    persistent uDaUnlim uQaUnlim 
    persistent uDaPI uQaPI
 if isempty(ydInt)
    ydInt = single(0);
    yqInt = single(0);
 end
    
 if(PIReset == 0)
    % new ramp calculation
		% correct calc
 
    iDaDes = TQC_IsdDes;
	iQaDes = TQC_IsqDes;
	

	iDaErrTust = (iDaDes - ISM_Isd)/2;
	iQaErrTust = (iQaDes - ISM_Isq)/2;
	
	omSttr = TQC_omSttr;
	agDelta = TQC_dtIsctl_Cc*omSttr*Decoup_coef;
	

	facIntglDaQa 	= TQC_kidq*TQC_dtIsctl_Cc;
	facIntglDa  	= TQC_kpd*agDelta;
	facIntglQa  	= TQC_kpq*agDelta;

	ydAdd	= facIntglDaQa*iDaErrTust - facIntglQa*iQaErrTust;
	yqAdd 	= facIntglDaQa*iQaErrTust + facIntglDa*iDaErrTust;

	ydInt   = ydInt + ydAdd;				
	yqInt   = yqInt + yqAdd;				
	
	yPd     = TQC_kpd*iDaErrTust*2;
	yPq     = TQC_kpq*iQaErrTust*2;
	yRvd    = TQC_Rv*ISM_Isd;
	yRvq    = TQC_Rv*ISM_Isq;
	
    ydPFF = yPd - yRvd;
	yqPFF = yPq - yRvq + TQC_UsqFluxExc;

	% calulation of feed forward voltage
% 	uR 			= TQC_RSttrFdFwd_Cc*iDaDesIntrpn;
% 	rIndu 		= omSttr*TQC_LQaFdFwd_Cc;
% 	uL 			= rIndu*iQaDesIntrpn;
% 	uDaFdFwd	= uR - uL;
% 	
% 	uR 			= TQC_RSttrFdFwd_Cc*iQaDesIntrpn;
% 	rIndu 		= omSttr*TQC_LDaFdFwd_Cc;
% 	uL 			= rIndu*iDaDesIntrpn;
% 	uQaFdFwd 	= uR + uL;
	
% 	if(TQC_bUseUFwdLimn_Cc)
%         % add uFdFwd before limitation
% 		ydPFF = ydPFF + uDaFdFwd;
% 		yqPFF = yqPFF + uQaFdFwd;
% 	end
	
	uDaUnlim = ydInt + ydPFF;		 
	uQaUnlim = yqInt + yqPFF;		
	
	
    if(uDaUnlim > TQC_uDaMax_Cc)
		uDaPI 		= TQC_uDaMax_Cc;
		ydInt 		= uDaPI - ydPFF;	
    else
        if(uDaUnlim < -TQC_uDaMax_Cc)
            uDaPI 	= -TQC_uDaMax_Cc;
			ydInt 	= uDaPI - ydPFF;	
        else	
			uDaPI 	= uDaUnlim;
			ydInt 	= ydInt + ydAdd;			
        end
    end


    if(uQaUnlim > TQC_uQaMax_Cc)
		uQaPI		= TQC_uQaMax_Cc;
		yqInt 		= uQaPI - yqPFF;	
    else
        if(uQaUnlim < -TQC_uQaMax_Cc)
			uQaPI	= -TQC_uQaMax_Cc;
			yqInt	= uQaPI - yqPFF;	
        else	
			uQaPI	= uQaUnlim;
			yqInt	= yqInt + yqAdd;			
        end
    end
	
%     if(TQC_bUseUFwdLimn_Cc == 0)
%         % add uFdFwd after limitation
% 		uDaPI = uDaPI + uDaFdFwd;
% 		uQaPI = uQaPI + uQaFdFwd;
%     end

	TQC_UsdPI = uDaPI;
	TQC_UsqPI = uQaPI;
	
    % 	Debug 
 	facIntglDa_Dbg      = facIntglDa;
 	facIntglQa_Dbg      = facIntglQa;
 	facIntglDaQa_Dbg    = facIntglDaQa;
 	uDaUnlim_Dbg        = uDaUnlim;
 	uQaUnlim_Dbg        = uQaUnlim;
 	iDaDes_Dbg          = iDaDes;
 	iQaDes_Dbg          = iQaDes;
% 	uDaFdFwd_Dbg        = uDaFdFwd;
% 	uQaFdFwd_Dbg        = uQaFdFwd;

else 
	ydInt	= single(0);
	yqInt	= single(0);
	TQC_UsdPI = single(0);
	TQC_UsqPI = single(0);
    facIntglDa_Dbg = single(0);
    facIntglQa_Dbg = single(0);
    facIntglDaQa_Dbg = single(0);
    uDaUnlim_Dbg = single(0);
    uQaUnlim_Dbg = single(0);
    iDaDes_Dbg = single(0);
    iQaDes_Dbg = single(0); 
 end

== stateflow chart MDCC_DeadComp/DoCurCtr_sys/MDCC/SVM_Calc/DeadTime_Compensation/Chart1 ==
  (default) -> (junction 11)
  (junction 11) -> (junction 13) [order 1] : [(Trq_IN>=Trq_High)]
      | {
      |    ReduOut =single(1);
      | }
  (junction 11) -> (junction 19) [order 3]
  (junction 11) -> (junction 14) [order 2] : [(Trq_IN<Trq_Low)]
      | {
      |    ReduOut =single(0);
      | }
  (junction 13) -> (junction 22)
  (junction 19) -> (junction 21) : {
      | ReduOut =ReduOut_Pre;
      | }
  (junction 21) -> (junction 14)
  (junction 22) -> (junction 14)
  data: ReduOut output single; Trq_Low input single; Trq_High input single; Trq_IN input single; ReduOut_Pre input single
